simulink model "Electromech_sys_current"  (R2025b)
settings: Solver=VariableStepAuto  StartTime=0.0  StopTime=10.0  RelTol=1e-3
values from neighbouring files (symbols this model uses):
  p_0 = 0    [Init_Simulink_param_nl_Electromech.m]
  phat_0 = 1e-3    (= 0.001)    [Init_Simulink_param_nl_Electromech.m]
  q_0 = 0    [Init_Simulink_param_nl_Electromech.m]
  Q_0 = 0    [Init_Simulink_param_nl_Electromech.m]
  qhat_0 = 2e-4    (= 0.0002)    [Init_Simulink_param_nl_Electromech.m]
  Qhat_0 = 5e-8    (= 5e-08)    [Init_Simulink_param_nl_Electromech.m]
undefined symbols (not defined in the file or in its folder): params
settings Model: Creator=filippougolini  LastModifiedBy=filippougolini

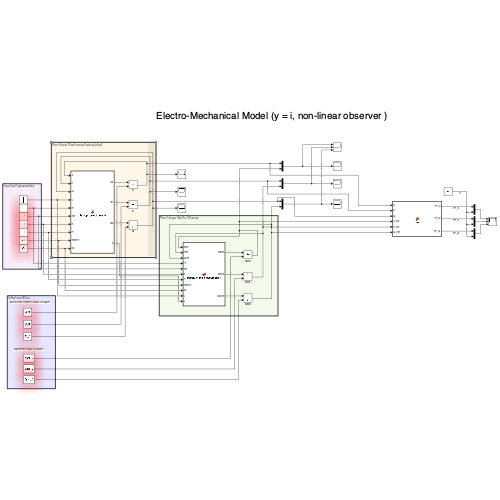
[thumbnail: Simulink's stored preview of the top-level diagram]
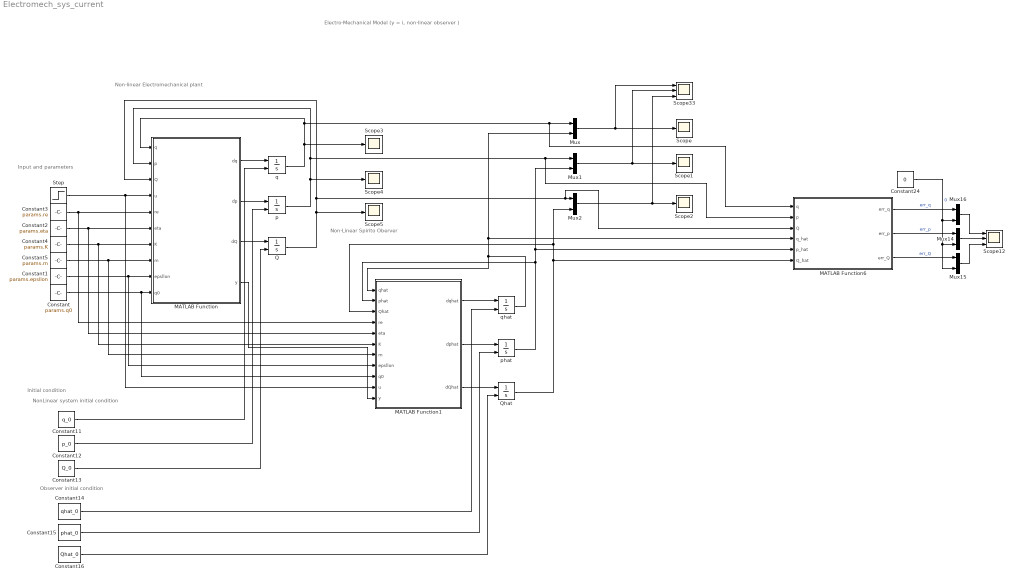
== system Electromech_sys_current ==
  note: Input and parameters
  note: NonLinear system initial condition
  note: Non-linear Electromechanical plant
  note: Non-Linear Spirito Oberver
  note: Electro-Mechanical Model (y = i, non-linear observer )
  note: Initial condition
  note: Observer initial condition
  Constant : Constant  Value=params.q0
  Constant1 : Constant  Value=params.epsllon
  Constant11 : Constant  Value=q_0
  Constant12 : Constant  Value=p_0
  Constant13 : Constant  Value=Q_0
  Constant14 : Constant  Value=qhat_0
  Constant15 : Constant  Value=phat_0
  Constant16 : Constant  Value=Qhat_0
  Constant2 : Constant  Value=params.eta
  Constant24 : Constant  Value=0
  Constant3 : Constant  Value=params.re
  Constant4 : Constant  Value=params.K
  Constant5 : Constant  Value=params.m
  MATLAB Function : MATLAB Function  TreatAsAtomicUnit=on
  MATLAB Function1 : MATLAB Function  TreatAsAtomicUnit=on
  MATLAB Function6 : MATLAB Function  TreatAsAtomicUnit=on
  Mux{,1..2,14..16} (6 alike) : Mux  Inputs=2
  Q : Integrator  InitialConditionSource=external
  Qhat : Integrator  InitialConditionSource=external  InitialCondition=30e-9
  Scope{,1..5} (6 alike) : Scope
      Scope settings: ActiveDisplayYMinimum=-4.4929456410290065E-5  ActiveDisplayYMaximum=0.00036894675529116814
      Scope1 settings: ActiveDisplayYMinimum=-1  ActiveDisplayYMaximum=1
      Scope2 settings: ActiveDisplayYMinimum=-1  ActiveDisplayYMaximum=1  DataLoggingVariableName=ScopeData2
      Scope3 settings: ActiveDisplayYMinimum=-4.0944874698701246E-5  ActiveDisplayYMaximum=0.0003685038722883113  DataLoggingVariableName=ScopeData3
      Scope4 settings: ActiveDisplayYMinimum=-1  ActiveDisplayYMaximum=1  DataLoggingVariableName=ScopeData4
      Scope5 settings: ActiveDisplayYMinimum=-1  ActiveDisplayYMaximum=1  DataLoggingVariableName=ScopeData5
  Scope12 : Scope  NumInputPorts=3
      settings: ActiveDisplayYMinimum=-0.00022777115343680583  ActiveDisplayYMaximum=2.90672954688174E-5  DataLoggingVariableName=ScopeData12
  Scope33 : Scope  NumInputPorts=3
      settings: ActiveDisplayString=3  ActiveDisplayYMinimum=-7.4244254076098763E-9  ActiveDisplayYMaximum=5.638049171195665E-8  DataLoggingVariableName=ScopeData33
  Step : Step  After=5e3  SampleTime=0
  p : Integrator  InitialConditionSource=external
  phat : Integrator  InitialConditionSource=external  InitialCondition=5e-4
  q : Integrator  InitialConditionSource=external
  qhat : Integrator  InitialConditionSource=external  InitialCondition=20e-5
  wires:
  Mux16/1 -> Scope12/1
  Constant5/1 -> MATLAB Function/8(m), MATLAB Function1/7(m)
  Mux1/1 -> Scope33/2, Scope1/1
  Mux/1 -> Scope33/1, Scope/1
  Mux14/1 -> Scope12/2
  Constant13/1 -> Q/2
  phat/1 -> MATLAB Function6/5(p_hat), Mux1/2, MATLAB Function1/2(phat)
  Step/1 -> MATLAB Function1/10(u), MATLAB Function/4(u)
  Constant14/1 -> qhat/2
  Constant24/1 -> Mux15/2, Mux14/2, Mux16/2  "0"
  Constant12/1 -> p/2
  p/1 -> Scope4/1, Mux1/1, MATLAB Function6/2(p), MATLAB Function/2(p)
  MATLAB Function1/2(dphat) -> phat/1
  Mux2/1 -> Scope33/3, Scope2/1
  Mux15/1 -> Scope12/3
  Constant3/1 -> MATLAB Function/5(re), MATLAB Function1/4(re)
  Constant1/1 -> MATLAB Function/9(epsllon), MATLAB Function1/8(epsllon)
  Constant/1 -> MATLAB Function1/9(q0), MATLAB Function/10(q0)
  qhat/1 -> MATLAB Function1/1(qhat), Mux/2, MATLAB Function6/4(q_hat)
  q/1 -> Scope3/1, MATLAB Function/1(q), Mux/1, MATLAB Function6/1(q)
  Constant15/1 -> phat/2
  Qhat/1 -> MATLAB Function6/6(Q_hat), Mux2/2, MATLAB Function1/3(Qhat)
  MATLAB Function/3(dQ) -> Q/1
  MATLAB Function/1(dq) -> q/1
  MATLAB Function6/3(err_Q) -> Mux15/1  "err_Q"
  MATLAB Function/2(dp) -> p/1
  MATLAB Function/4(y) -> MATLAB Function1/11(y)
  Q/1 -> Mux2/1, MATLAB Function6/3(Q), MATLAB Function/3(Q), Scope5/1
  Constant2/1 -> MATLAB Function/6(eta), MATLAB Function1/5(eta)
  MATLAB Function1/3(dQhat) -> Qhat/1
  Constant16/1 -> Qhat/2
  Constant4/1 -> MATLAB Function/7(K), MATLAB Function1/6(K)
  MATLAB Function1/1(dqhat) -> qhat/1
  MATLAB Function6/2(err_p) -> Mux14/1  "err_p"
  Constant11/1 -> q/2
  MATLAB Function6/1(err_q) -> Mux16/1  "err_q"

== matlab function Electromech_sys_current/MATLAB Function1 ==
  data: qhat input; phat input; Qhat input; re input; eta input; K input; m input; epsllon input; q0 input; u input; dqhat output; y input; dphat output; dQhat output
function [dqhat, dphat, dQhat] = observer_pH_electromech_i(qhat, phat, Qhat, ...
    re, eta, K, m, epsllon, q0, u, y)

    % Port-Hamiltonian structure matrices
    J = [  0  1  0;
          -1  0  0;
           0  0  0 ];

    R = diag([0, eta, 1/re]);
    g = [0; 0; 1/re];

    % -------- Hamiltonian gradient at xhat = [qhat; phat; Qhat] --------
    Cqh    = epsllon * (qhat + q0)^4;

    % dH/dqhat
    dHhdqh = K*qhat - 2*Qhat^2 / (epsllon * (qhat + q0)^5);
    % dH/dphat
    dHhdph = phat / m;
    % dH/dQhat
    dHhdQh = Qhat / Cqh;

    gradHh = [dHhdqh; dHhdph; dHhdQh];
    
    % -------- Observer gain L --------
    gamma = 20;
    L  = gamma * g;
    Lcol = -L.';       % ensure it's 3x1

    yhat =  - (1/re) * dHhdQh + (1/re) * u;

    % -------- Observer dynamics --------
    % Note: J and R are constant
    xhatdot = (J - R) * gradHh + g*u + Lcol * (y - yhat);

    dqhat = xhatdot(1);
    dphat = xhatdot(2);
    dQhat = xhatdot(3);
end

== matlab function Electromech_sys_current/MATLAB Function ==
  data: q input; p input; Q input; u input; dq output; re input; eta input; K input; m input; epsllon input; q0 input; dp output; dQ output; y output
function [dq, dp, dQ, y] = plant_pH_electromech(q, p, Q, u, re, eta, K, m, epsllon, q0)
% Electro-mechanical pH plant

    % Parameters: m, K, eta, eps, re, q0 in workspace

    J = [  0  1  0;
          -1  0  0;
           0  0  0 ];

    R = diag([0, eta, 1/re]);
    g = [0; 0; 1/re];

    % Hamiltonian gradient gradH(q,p,Q)
    Cq   = epsllon * (q + q0)^4;

    dHdq = K*q - 2*Q^2 / (epsllon * (q + q0)^5);
    dHdp = p / m;
    dHdQ = Q / Cq;

    gradH = [dHdq; dHdp; dHdQ];

    xdot = (J - R) * gradH + g*u;

    y = - (1/re) * dHdQ + (1/re) * u; % i = Q_dot
    
    dq = xdot(1);
    dp = xdot(2);
    dQ = xdot(3);
end

== matlab function Electromech_sys_current/MATLAB Function6 ==
  data: q input; err_q output; p input; Q input; q_hat input; p_hat input; Q_hat input; err_p output; err_Q output
function [err_q, err_p, err_Q] = error(q, p, Q, q_hat, p_hat, Q_hat)

    err_q = q - q_hat;
    err_p = p - p_hat;
    err_Q = Q - Q_hat;
end
